simulink model "Models"  (R2020a)
settings: Solver=FixedStepAuto  StartTime=0.0  StopTime=10  MaxStep=tStepMax  RelTol=1e-3
values from neighbouring files (symbols this model uses):
  c = app.cNmradsEditField.Value    [Feedforward_app_exported.m]    (also in app2_exported.m; init1.m = 0.5)
  g = 9.8    [Feedforward_app_exported.m]    (also in app2_exported.m; init1.m = 10)
  L = app.LmEditField.Value    [Feedforward_app_exported.m]    (also in app2_exported.m; init1.m = 1)
  m = app.massekgEditField.Value    [Feedforward_app_exported.m]    (also in app2_exported.m; init1.m = 1)
  theta0 = 0    [Feedforward_app_exported.m]    (also in app2_exported.m; init1.m = 0.10471975512)
  thetadot0 = 0    [Feedforward_app_exported.m]    (also in app2_exported.m; init1.m)
settings Model: Creator=hussein  LastModifiedBy=hussein
settings DataIOCC: SaveOutput=off  SignalLogging=off  DSMLogging=off  ReturnWorkspaceOutputs=off

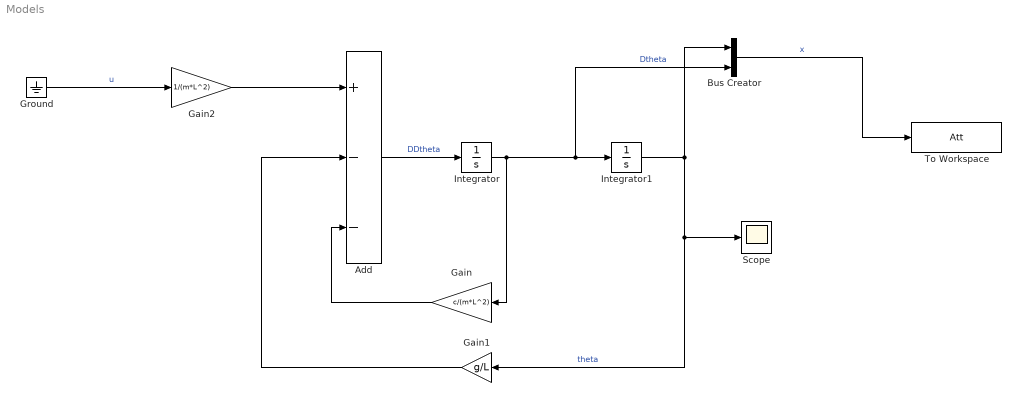
== system Models ==
  Add : Sum  Inputs=+--
  Bus Creator : BusCreator  Inputs=2
  Gain : Gain  Gain=c/(m*L^2)
  Gain1 : Gain  Gain=g/L
  Gain2 : Gain  Gain=1/(m*L^2)
  Ground : Ground
  Integrator : Integrator  InitialCondition=thetadot0
  Integrator1 : Integrator  InitialCondition=theta0
  Scope : Scope
  To Workspace : ToWorkspace  VariableName=Att  SaveFormat=Timeseries  SampleTime=-1
  wires:
  Ground/1 -> Gain2/1  "u"
  Add/1 -> Integrator/1  "DDtheta"
  Integrator/1 -> Gain/1, Bus Creator/2, Integrator1/1  "Dtheta"
  Gain/1 -> Add/3
  Integrator1/1 -> Bus Creator/1, Gain1/1, Scope/1  "theta"
  Gain1/1 -> Add/2
  Gain2/1 -> Add/1
  Bus Creator/1 -> To Workspace/1  "x"
